simulink library "GroupLib"  (R2012b)
settings: Solver=ode45  StartTime=0.0  StopTime=10.0  RelTol=1e-3
settings Model: Creator=higashit  LastModifiedBy=higashit

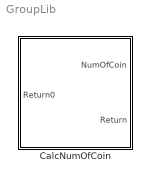
== system GroupLib ==
  CalcNumOfCoin : Subsystem  mask{Coin=500}
      mask prompts: Coin "硬貨の価格"

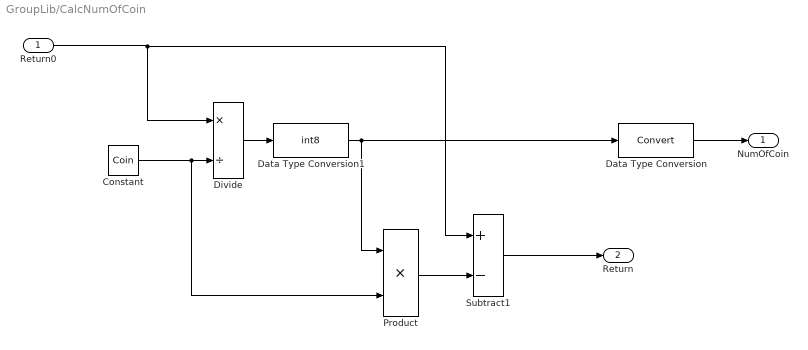
== system GroupLib/CalcNumOfCoin ==
  Return0 : Inport
  Constant : Constant  Value=Coin
  Data Type Conversion : DataTypeConversion
  Data Type Conversion1 : DataTypeConversion  OutDataTypeStr=int8
  Divide : Product  Inputs=*/  OutDataTypeStr=int8
  Product : Product  RndMeth=Zero
  Subtract1 : Sum  Inputs=+-
  NumOfCoin : Outport
  Return : Outport  Port=2
  wires:
  Constant/1 -> Product/2, Divide/2
  Product/1 -> Subtract1/2
  Data Type Conversion/1 -> NumOfCoin/1
  Divide/1 -> Data Type Conversion1/1
  Subtract1/1 -> Return/1
  Return0/1 -> Divide/1, Subtract1/1
  Data Type Conversion1/1 -> Product/1, Data Type Conversion/1
